simulink subsystem "AirData"  (R2024b)
settings: Solver=VariableStepAuto  StartTime=0.0  StopTime=10.0  RelTol=1e-3
libraries: aerolibasang x2, aerolibatmos2 x1
settings Model: Creator=thesa  LastModifiedBy=jack

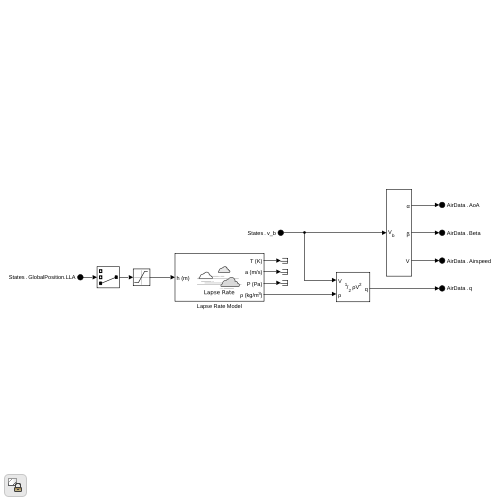
[thumbnail: Simulink's stored preview of the top-level diagram]
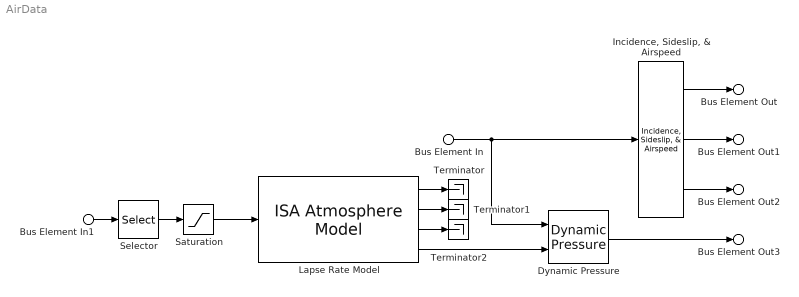
== system AirData ==
  Bus Element In : Inport  PortName=States  Element=v_b
  Bus Element In1 : Inport  PortName=States  Element=GlobalPosition.LLA
  Dynamic Pressure : aerolibasang/Dynamic Pressure
  "Incidence, Sideslip, & Airspeed" : aerolibasang/Incidence, Sideslip, & Airspeed
  Lapse Rate Model : aerolibatmos2/ISA Atmosphere Model  useExtended=off  action=Warning  custom=on  viscosityOut=off  g=9.80665  gamma=1.4  R=287.0531  L=0.0065  h_trop=11000  h_strat=20000  rho0=1.225  P0=101325  T0=288.15  h0=0  S=110.4  Tref=273.15  muref=1.716e-5
  Saturation : Saturate  UpperLimit=20000  LowerLimit=0
  Selector : Selector  InputPortWidth=3  IndexOptions=Index vector (dialog)  Indices=3  OutputSizes=1
  Terminator : Terminator
  Terminator1 : Terminator
  Terminator2 : Terminator
  Bus Element Out : Outport  PortName=AirData  Element=AoA
  Bus Element Out1 : Outport  PortName=AirData  Element=Beta
  Bus Element Out2 : Outport  PortName=AirData  Element=Airspeed
  Bus Element Out3 : Outport  PortName=AirData  Element=q
  wires:
  "Incidence, Sideslip, & Airspeed"/1 -> Bus Element Out/1
  "Incidence, Sideslip, & Airspeed"/2 -> Bus Element Out1/1
  "Incidence, Sideslip, & Airspeed"/3 -> Bus Element Out2/1
  Bus Element In/1 -> "Incidence, Sideslip, & Airspeed"/1, Dynamic Pressure/1
  Lapse Rate Model/4 -> Dynamic Pressure/2
  Dynamic Pressure/1 -> Bus Element Out3/1
  Bus Element In1/1 -> Selector/1
  Selector/1 -> Saturation/1
  Saturation/1 -> Lapse Rate Model/1
  Lapse Rate Model/1 -> Terminator/1
  Lapse Rate Model/2 -> Terminator1/1
  Lapse Rate Model/3 -> Terminator2/1
